simulink model "PID_CONTROLLER_Harness1"  (R2021b)
settings: Solver=FixedStepAuto  StartTime=0.0  StopTime=10  RelTol=1e-3
undefined symbols (not defined in the file): sigbuilder_block
settings Model: Creator=sudhir  LastModifiedBy=sudhir
settings DataIOCC: SaveOutput=off  SaveTime=off

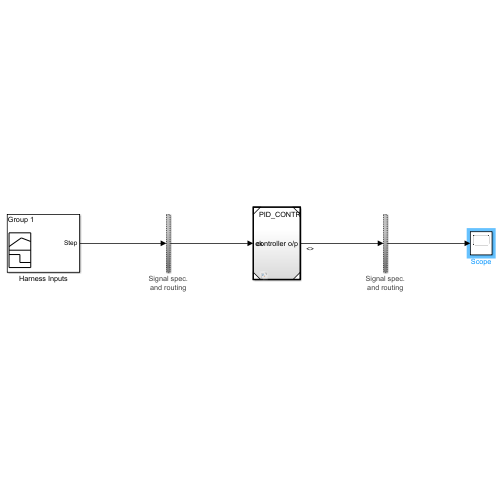
[thumbnail: Simulink's stored preview of the top-level diagram]
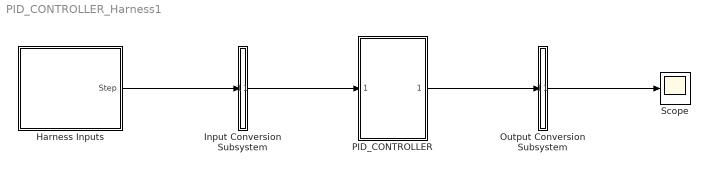
== system PID_CONTROLLER_Harness1 ==
  Harness Inputs : Subsystem  Tag=STV Subsys  LoadFcn=sigbuilder_block('load');  StartFcn=sigbuilder_block('start');  StopFcn=sigbuilder_block('stop');  ClipboardFcn=sigbuilder_block('clipboard');  mask(Sigbuilder block){tuvar=[0:10]}
      mask init:
      | if ~strcmp(get_param(bdroot(gcb),'SimulationStatus'),'stopped'),tuvar = sigbuilder_block('maskInit'); end
      settings: CopyFcn=sigbuilder_block('copy');  DeleteFcn=sigbuilder_block('delete');  ModelCloseFcn=sigbuilder_block('modelClose');  PreSaveFcn=sigbuilder_block('preSave');  PauseFcn=sigbuilder_block('pause');  ContinueFcn=sigbuilder_block('continue');  NameChangeFcn=sigbuilder_block('namechange');  OpenFcn=sigbuilder_block('open',[50 50 520 400 ]);  CloseFcn=sigbuilder_block('close');
      mask Display: plot(0, 0, 100, 100,[2, 2, 32, 32, 2], [68, 8, 8, 68, 68],[32, 2], [38, 38], [32, 19, 2],[53, 60, 44], [32, 17, 17, 2],[16, 16, 31, 31]);txt = getActiveGroup(gcbh);text(2, 100, txt,'verticalAlignment', 'top');
  Input Conversion Subsystem : Subsystem  Tag=__SLT_ICS__  Description=|
      | Signal spec.
      | and routing
      settings: AttributesFormatString=%<Description>
  Output Conversion Subsystem : Subsystem  Tag=__SLT_OCS__  Description=|
      | Signal spec.
      | and routing
      settings: AttributesFormatString=%<Description>
  PID_CONTROLLER : ModelReference  ModelNameDialog=PID_CONTROLLER  SimulationMode=Normal  ModelReferenceVersion=1.42
  Scope : Scope
  wires:
  Harness Inputs/1(Step) -> Input Conversion Subsystem/1(Inport_1)
  Output Conversion Subsystem/1(Outport_1) -> Scope/1
  Input Conversion Subsystem/1(Outport_1) -> PID_CONTROLLER/1
  PID_CONTROLLER/1 -> Output Conversion Subsystem/1(Inport_1)

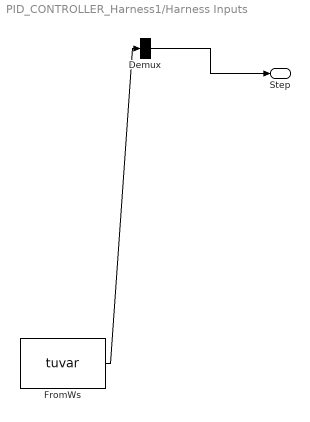
== system PID_CONTROLLER_Harness1/Harness Inputs ==
  Demux : Demux  Tag=STV Demux  Outputs=1
  FromWs : FromWorkspace  Tag=STV FromWs  VariableName=tuvar
      SigBuilderData=|
      | dataSet.timeRange = [0 1]
      | dataSet.name = 'Group 1'
      | sbobj.Name = 'Signal Builder'
      | sbobj.Groups.Name = 'Group 1'
      | sbobj.Groups.Signals.Name = 'Step'
      | sbobj.Groups.Signals.XData = [0 0.5 0.5 1]
      | sbobj.Groups.Signals.YData = [0 0 1 1]
      | sbobj.Groups.TimeRange = [0 1]
  Step : Outport  Tag=STV Outport
  wires:
  FromWs/1 -> Demux/1
  Demux/1 -> Step/1

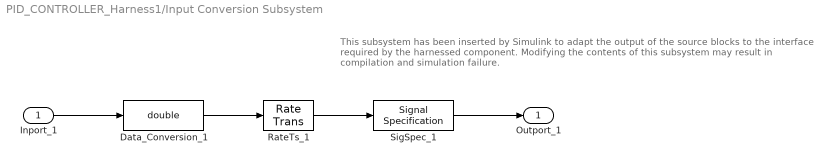
== system PID_CONTROLLER_Harness1/Input Conversion Subsystem ==
  note: This subsystem has been inserted by Simulink to adapt the output of the source blocks to the interface required by the harnessed component.
      |  Modifying the contents of this subsystem may result in compilation and simulation failure.
  Inport_1 : Inport
  Data_Conversion_1 : DataTypeConversion  OutDataTypeStr=double  SaturateOnIntegerOverflow=on  RndMeth=Zero
  RateTs_1 : RateTransition  OutPortSampleTime=0.01
  SigSpec_1 : SignalSpecification  OutDataTypeStr=double  Dimensions=[1]  SampleTime=0.01
  Outport_1 : Outport
  wires:
  SigSpec_1/1 -> Outport_1/1
  RateTs_1/1 -> SigSpec_1/1
  Data_Conversion_1/1 -> RateTs_1/1
  Inport_1/1 -> Data_Conversion_1/1

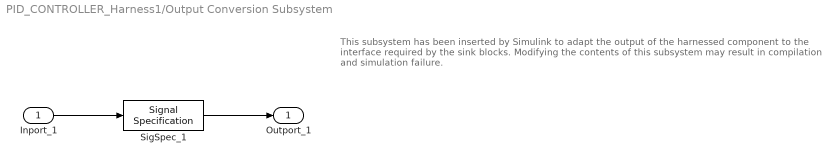
== system PID_CONTROLLER_Harness1/Output Conversion Subsystem ==
  note: This subsystem has been inserted by Simulink to adapt the output of the harnessed component to the interface required by the sink blocks.
      |  Modifying the contents of this subsystem may result in compilation and simulation failure.
  Inport_1 : Inport
  SigSpec_1 : SignalSpecification  OutDataTypeStr=double  Dimensions=[1]  SampleTime=0.01
  Outport_1 : Outport
  wires:
  Inport_1/1 -> SigSpec_1/1
  SigSpec_1/1 -> Outport_1/1
